simulink model "rcosine"  (R2021a)
settings: Solver=FixedStepDiscrete  StartTime=0.0  StopTime=10.0  RelTol=1e-3
libraries: dspmlti4 x2
settings Model: Creator=ishaanagarwal  LastModifiedBy=MichaelWu
settings OptimizationCC: BlockReduction=off  ConditionallyExecuteInputs=off
settings DebuggingCC: InheritedTsInSrcMsg=none  SingleTaskRateTransMsg=error

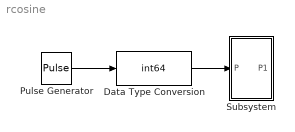
== system rcosine ==
  Data Type Conversion : DataTypeConversion  OutDataTypeStr=int64
  Pulse Generator : DiscretePulseGenerator  Period=10  PulseWidth=5
  Subsystem : Subsystem
  wires:
  Data Type Conversion/1 -> Subsystem/1(P)
  Pulse Generator/1 -> Data Type Conversion/1

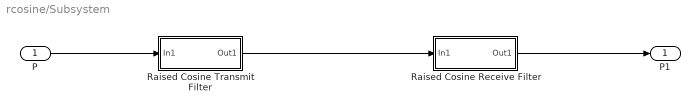
== system rcosine/Subsystem ==
  P : Inport  OutDataTypeStr=int64  PortDimensions=1
  Raised Cosine Receive Filter : Subsystem  mask(Raised Cosine Receive Filter){filtType=Square root, R=double(0.2), filtSpan=double(10), N=double(8), downFactor=double(8), downOffset=double(0), filterGain=double(1), InputProcessing=Elements as channels (sample based), RateOptions=Allow multirate processing, framing=Mute, checkCoeff=off, variableName=rcRxFilt, currentFiltSpan=double(10), D=double(5), inputOffset=double(0), sampMode=Mute, saveAsFlag=double(0), rateMode=Downsampling, checkGain=Normalized, launchFVT=on, roundingMode=Floor, overflowMode=off, coeffMode=Specify word length, coeffWordLength=double(16), coeffFracLength=double(15), coeffDataTypeStr=fixdt(1,16), coeffMin=[], coeffMax=[], coeffLastDataTypeStr=fixdt(1,16), prodOutputMode=Binary point scaling, prodOutputWordLength=double(16), prodOutputFracLength=double(0), prodOutputDataTypeStr=fixdt(1,16,0), prodOutputLastDataTypeStr=fixdt(1,16,0), accumMode=Binary point scaling, accumWordLength=double(16), accumFracLength=double(0), accumDataTypeStr=fixdt(1,16,0), accumLastDataTypeStr=fixdt(1,16,0), outputMode=Binary point scaling, outputWordLength=double(16), outputFracLength=double(0), outputDataTypeStr=fixdt(1,16,0), outputMin=[], outputMax=[], outputLastDataTypeStr=fixdt(1,16,0), LockScale=off}
      mask prompts: filtType "Filter shape:"; R "Rolloff factor:"; filtSpan "Filter span in symbols:"; N "Input samples per symbol:"; downFactor "Decimation factor:"; downOffset "Decimation offset:"; filterGain "Linear amplitude filter gain:"; InputProcessing "dsp:FIRMultirateBlockDialog:InputProc_MP"; RateOptions "dsp:FIRMultirateBlockDialog:RateOptions_MP"; checkCoeff "Export filter coefficients to workspace"; variableName "Coefficient variable name:"; currentFiltSpan "Current filter span in symbols:"; D "Group delay (number of symbols):"; sampMode "Input sampling mode:"; saveAsFlag "Save_as flag:"; rateMode "Output mode:"; checkGain "Filter gain:"; launchFVT "Visualize filter with FVTool"; roundingMode "dspshared:FixptDialog:roundingMode"; overflowMode "Simulink:masks:SaturateOnIntegerOverflow_MP"; LockScale "dspshared:FixptDialog:lockAgnstChanges"
      mask help: Filter the input, and, if selected, downsample, using a normal or square root raised cosine FIR filter.
      mask init:
      | InputProcessing = double(2);
      | coeff = reshape(double([-0.006003286587616524 -0.005144225554935529 -0.0029018448367485235 0.00044150963068243236 0.004315735823570269 0.007946919193105199 0.01049533975797793 0.011225159585144306 0.009674451151703551 0.005790697043638924 -7.581652757135339e-18 -0.00681200565674492 -0.013414453134119732 -0.018429673666006872 -0.020587012602187465 -0.018989369401589986 -0.01334263000888136 -0.004099700124818936 0.0075184161679393525 0.01964330583622726 0.030016432938082625 0.036352558555173935 0.03675670126548123 0.030127294329476258 0.016474018654190382 -0.0029132831651865385 -0.02548868226937497 -0.04768274492821171 -0.06532584444022004 -0.07421175377365097 -0.07072455390393828 -0.05243631513297172 -0.01858152998446693 0.029672166134325467 0.08921038794281236 0.1552321703944631 0.22175972309238012 0.2823350081994533 0.33081031138933115 0.362123383225845 0.37294751443000096 0.362123383225845 0.33081031138933115 0.2823350081994533 0.22175972309238012 0.1552321703944631 0.08921038794281236 0.029672166134325467 -0.01858152998446693 -0.05243631513297172 -0.07072455390393828 -0.07421175377365097 -0.06532584444022004 -0.04768274492821171 -0.02548868226937497 -0.0029132831651865385 0.016474018654190382 0.030127294329476258 0.03675670126548123 0.036352558555173935 0.030016432938082625 0.01964330583622726 0.0075184161679393525 -0.004099700124818936 -0.01334263000888136 -0.018989369401589986 -0.020587012602187465 -0.018429673666006872 -0.013414453134119732 -0.00681200565674492 -7.581652757135339e-18 0.005790697043638924 0.009674451151703551 0.011225159585144306 0.01049533975797793 0.007946919193105199 0.004315735823570269 0.00044150963068243236 -0.0029018448367485235 -0.005144225554935529 -0.006003286587616524]).', [1  81]);
      | downFactor = double(8);
      | downOffset = double(0);
      | inputOffset = double(0);
      | outputMax = [];
      | outputMin = [];
      mask Help: eval('blocksethelp');
      mask TypeOptions filtType: Normal | Square root
      mask TypeOptions InputProcessing: Columns as channels (frame based) | Elements as channels (sample based)
      mask Callback InputProcessing: commblkrcfiltrx(gcbh,'cbInputProcessing');
      mask TypeOptions RateOptions: Enforce single-rate processing | Allow multirate processing
      mask TypeOptions framing: Enforce single-rate processing | Allow multirate processing | Maintain input frame rate | Maintain input frame size | Mute
      mask Callback checkCoeff: commblkrcfiltrx(gcbh,'cbCheckCoeff');
      mask Callback variableName: commblkrcfiltrx(gcbh,'dialogdynamic');
      mask TypeOptions sampMode: Frame-based | Sample-based | Mute
      mask TypeOptions rateMode: Downsampling | None
      mask TypeOptions checkGain: Normalized | User-specified
      mask TypeOptions roundingMode: Ceiling | Convergent | Floor | Nearest | Round | Simplest | Zero
      mask TypeOptions coeffMode: Same word length as input | Specify word length | Binary point scaling | Slope and bias scaling
      mask TypeOptions prodOutputMode: Same as input | Binary point scaling | Slope and bias scaling
      mask TypeOptions accumMode: Same as product output | Same as input | Binary point scaling | Slope and bias scaling
      mask TypeOptions outputMode: Same as accumulator | Same as input | Binary point scaling | Slope and bias scaling
      mask Display:
      | coeffs = rcosdesign(0.2, 10, 8, 'sqrt'); % default
      | % This plot does not change enough to make it worth updating to specifics
      | % Just use a representative plot for all cases.
      | %
      | %-- Init icon variables
      | %   (draw default icon in case of early returns,
      | %    e.g. due to errors from undefined mask params)
      | icon.str = get_param(gcbh,'filtType');
      | icon.x = 0.5;
      | icon.y = 0.25;
      | icon.plot = coeffs/max(coeffs)*0.40+0.50;
      | icon.xx = (1:length(coeffs))/length(coeffs);
      | 
      | plot(0,0,1,1,icon.xx,icon.plot);
      | text(icon.x,icon.y,icon.str,'horiz','center');
  Raised Cosine Transmit Filter : Subsystem  mask(Raised Cosine Transmit Filter){filtType=Square root, R=double(0.2), filtSpan=double(10), N=double(8), filterGain=double(1), InputProcessing=Elements as channels (sample based), RateOptions=Allow multirate processing, framing=Mute, checkCoeff=off, variableName=rcTxFilt, checkGain=Normalized, sampMode=Mute, saveAsFlag=double(0), currentFiltSpan=double(10), D=double(5), launchFVT=on, roundingMode=Floor, overflowMode=off, coeffMode=Specify word length, coeffWordLength=double(16), coeffFracLength=double(15), coeffDataTypeStr=Inherit: Same word length as input, coeffMin=[], coeffMax=[], coeffLastDataTypeStr=fixdt(1,16), prodOutputMode=Binary point scaling, prodOutputWordLength=double(16), prodOutputFracLength=double(0), prodOutputDataTypeStr=Inherit: Same as input, prodOutputLastDataTypeStr=fixdt(1,16,0), accumMode=Binary point scaling, accumWordLength=double(16), accumFracLength=double(0), accumDataTypeStr=Inherit: Same as input, accumLastDataTypeStr=fixdt(1,16,0), outputMode=Binary point scaling, outputWordLength=double(16), outputFracLength=double(0), outputDataTypeStr=Inherit: Same as input, outputMin=[], outputMax=[], outputLastDataTypeStr=fixdt(1,16,0), LockScale=off}
      mask prompts: filtType "Filter shape:"; R "Rolloff factor:"; filtSpan "Filter span in symbols:"; N "Output samples per symbol:"; filterGain "Linear amplitude filter gain:"; InputProcessing "dsp:FIRMultirateBlockDialog:InputProc_MP"; RateOptions "dsp:FIRMultirateBlockDialog:RateOptions_MP"; checkCoeff "Export filter coefficients to workspace"; variableName "Coefficient variable name:"; checkGain "Filter gain:"; sampMode "Input sampling mode:"; saveAsFlag "Save_as flag:"; currentFiltSpan "Current filter span in symbols:"; D "Group delay (number of symbols):"; launchFVT "Visualize filter with FVTool"; roundingMode "dspshared:FixptDialog:roundingMode"; overflowMode "Simulink:masks:SaturateOnIntegerOverflow_MP"; LockScale "dspshared:FixptDialog:lockAgnstChanges"
      mask help: Upsample and filter the input signal using a normal or square root raised cosine FIR filter.
      mask init:
      | InputProcessing = double(2);
      | coeff = reshape(double([-0.006003286587616524 -0.005144225554935529 -0.0029018448367485235 0.00044150963068243236 0.004315735823570269 0.007946919193105199 0.01049533975797793 0.011225159585144306 0.009674451151703551 0.005790697043638924 -7.581652757135339e-18 -0.00681200565674492 -0.013414453134119732 -0.018429673666006872 -0.020587012602187465 -0.018989369401589986 -0.01334263000888136 -0.004099700124818936 0.0075184161679393525 0.01964330583622726 0.030016432938082625 0.036352558555173935 0.03675670126548123 0.030127294329476258 0.016474018654190382 -0.0029132831651865385 -0.02548868226937497 -0.04768274492821171 -0.06532584444022004 -0.07421175377365097 -0.07072455390393828 -0.05243631513297172 -0.01858152998446693 0.029672166134325467 0.08921038794281236 0.1552321703944631 0.22175972309238012 0.2823350081994533 0.33081031138933115 0.362123383225845 0.37294751443000096 0.362123383225845 0.33081031138933115 0.2823350081994533 0.22175972309238012 0.1552321703944631 0.08921038794281236 0.029672166134325467 -0.01858152998446693 -0.05243631513297172 -0.07072455390393828 -0.07421175377365097 -0.06532584444022004 -0.04768274492821171 -0.02548868226937497 -0.0029132831651865385 0.016474018654190382 0.030127294329476258 0.03675670126548123 0.036352558555173935 0.030016432938082625 0.01964330583622726 0.0075184161679393525 -0.004099700124818936 -0.01334263000888136 -0.018989369401589986 -0.020587012602187465 -0.018429673666006872 -0.013414453134119732 -0.00681200565674492 -7.581652757135339e-18 0.005790697043638924 0.009674451151703551 0.011225159585144306 0.01049533975797793 0.007946919193105199 0.004315735823570269 0.00044150963068243236 -0.0029018448367485235 -0.005144225554935529 -0.006003286587616524]).', [1  81]);
      | outputMax = [];
      | outputMin = [];
      | rateFactor = double(8);
      mask Help: eval('blocksethelp');
      mask TypeOptions filtType: Normal | Square root
      mask TypeOptions InputProcessing: Columns as channels (frame based) | Elements as channels (sample based)
      mask Callback InputProcessing: commblkrcfilttx(gcbh,'cbInputProcessing');
      mask TypeOptions RateOptions: Enforce single-rate processing | Allow multirate processing
      mask TypeOptions framing: Enforce single-rate processing | Allow multirate processing | Maintain input frame rate | Maintain input frame size | Mute
      mask Callback checkCoeff: commblkrcfilttx(gcbh,'cbCheckCoeff');
      mask Callback variableName: commblkrcfilttx(gcbh,'dialogdynamic');
      mask TypeOptions checkGain: Normalized | User-specified
      mask TypeOptions sampMode: Frame-based | Sample-based | Mute
      mask TypeOptions roundingMode: Ceiling | Convergent | Floor | Nearest | Round | Simplest | Zero
      mask TypeOptions coeffMode: Same word length as input | Specify word length | Binary point scaling | Slope and bias scaling
      mask TypeOptions prodOutputMode: Inherit via internal rule | Same as input | Binary point scaling | Slope and bias scaling
      mask TypeOptions accumMode: Inherit via internal rule | Same as product output | Same as input | Binary point scaling | Slope and bias scaling
      mask TypeOptions outputMode: Same as accumulator | Same as product output | Same as input | Binary point scaling | Slope and bias scaling
      mask Display:
      | coeffs = rcosdesign(0.2, 10, 8, 'sqrt'); % default
      | % This plot does not change enough to make it worth updating to specifics
      | % Just use a representative plot for all cases.
      | %
      | %-- Init icon variables
      | %   (draw default icon in case of early returns,
      | %    e.g. due to errors from undefined mask params)
      | icon.str = get_param(gcbh,'filtType');
      | icon.x = 0.5;
      | icon.y = 0.25;
      | icon.plot = coeffs/max(coeffs)*0.40+0.50;
      | icon.xx = (1:length(coeffs))/length(coeffs);
      | 
      | plot(0,0,1,1,icon.xx,icon.plot);
      | text(icon.x,icon.y,icon.str,'horiz','center');
  P1 : Outport  OutDataTypeStr=int64  SampleTime=1
  wires:
  Raised Cosine Transmit Filter/1(Out1) -> Raised Cosine Receive Filter/1(In1)
  Raised Cosine Receive Filter/1(Out1) -> P1/1
  P/1 -> Raised Cosine Transmit Filter/1(In1)

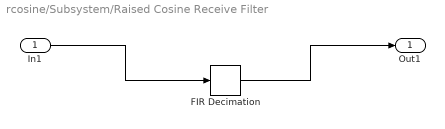
== system rcosine/Subsystem/Raised Cosine Receive Filter ==
  In1 : Inport  OutDataTypeStr=fixdt(1, 64, 0)  PortDimensions=1  SampleTime=0.125  LockScale=on
  FIR Decimation : dspmlti4/FIR Decimation  FilterSource=Dialog parameters  h=coeff  D=downFactor  filtStruct=Direct form  FilterObject=Hm_firdecim  framing=Allow multirate processing  inputOffset=(downFactor-downOffset)  outputBufInitCond=0  roundingMode=Floor  overflowMode=off  firstCoeffDataTypeStr=Inherit: Same word length as input  firstCoeffMin=[]  firstCoeffMax=[]  firstCoeffLastDataTypeStr=Inherit: Same word length as input  accumDataTypeStr=Inherit: Same as product output  accumLastDataTypeStr=Inherit: Same as product output  outputDataTypeStr=Inherit: Same as accumulator  outputMin=[]  outputMax=[]  outputLastDataTypeStr=Inherit: Same as accumulator
  Out1 : Outport  SampleTime=1
  wires:
  In1/1 -> FIR Decimation/1
  FIR Decimation/1 -> Out1/1

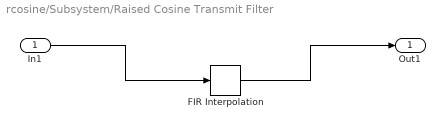
== system rcosine/Subsystem/Raised Cosine Transmit Filter ==
  In1 : Inport  OutDataTypeStr=int64  SampleTime=1
  FIR Interpolation : dspmlti4/FIR Interpolation  FilterSource=Dialog parameters  PrivateCoeffs=0  h=coeff  L=rateFactor  FilterObject=Hm_firinterp  framing=Allow multirate processing  outputBufInitCond=0  roundingMode=Floor  overflowMode=off  firstCoeffDataTypeStr=Inherit: Same word length as input  firstCoeffMin=[]  firstCoeffMax=[]  firstCoeffLastDataTypeStr=Inherit: Same word length as input  accumDataTypeStr=Inherit: Same as product output  accumLastDataTypeStr=Inherit: Same as product output  outputDataTypeStr=Inherit: Same as accumulator  outputMin=[]  outputMax=[]  outputLastDataTypeStr=Inherit: Same as accumulator
  Out1 : Outport  SampleTime=0.125
  wires:
  In1/1 -> FIR Interpolation/1
  FIR Interpolation/1 -> Out1/1
